simulink model "inverse_test"  (R2020b)
settings: Solver=VariableStepAuto  StartTime=0.0  StopTime=30  RelTol=1e-3
model workspace (MAT data in the model file):
  l1 = Simulink.Parameter
  l1.Value = 0.2
  l1.Description = '"Bicep length"'
  l1.DataType = 'auto'
  l1.Dimensions = [1 1]
  l2 = Simulink.Parameter
  l2.Value = 0.15
  l2.Description = '"Forearm length"'
  l2.DataType = 'auto'
  l2.Dimensions = [1 1]
libraries: pid_lib x2, simulink_extras x1
settings Model: PacingRate=0.500000  OrderedModelArguments=off  Creator=Luke Bidulka  LastModifiedBy=ndroz

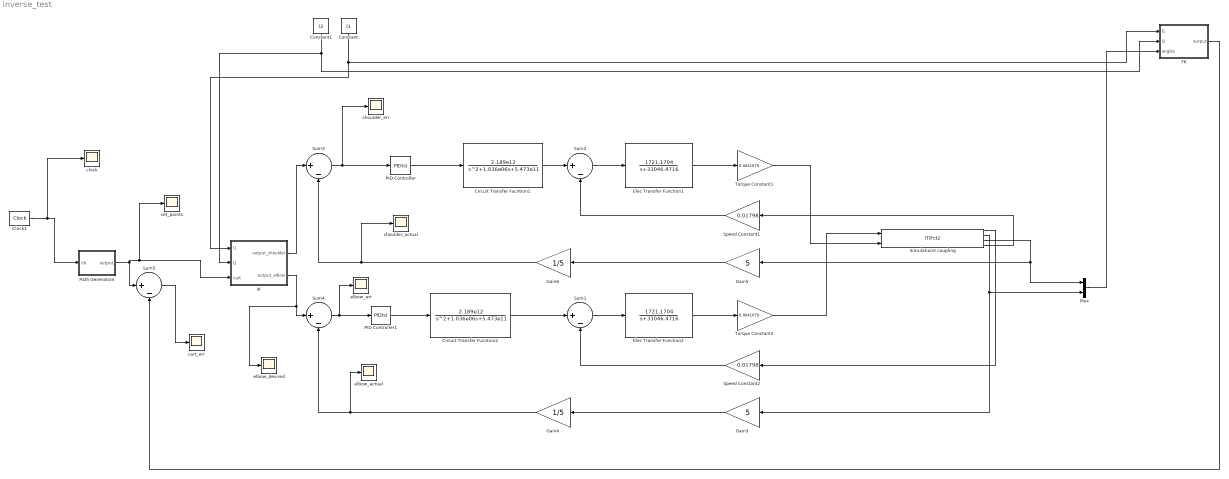
== system inverse_test ==
  Circuit Transfer Fucntion1 : TransferFcn  Numerator=[2.189e12]  Denominator=[1 1.036e06 5.473e11]
  Circuit Transfer Fucntion2 : TransferFcn  Numerator=[2.189e12]  Denominator=[1 1.036e06 5.473e11]
  Clock1 : simulink_extras/Flip Flops/Clock  period=0.01
  Constant : Constant  Value=l1
  Constant1 : Constant  Value=l2
  Elec Transfer Function1 : TransferFcn  Numerator=[1721.1704]  Denominator=[1 33046.4716]
  Elec Transfer Function2 : TransferFcn  Numerator=[1721.1704]  Denominator=[1 33046.4716]
  FK : MATLAB Function  TreatAsAtomicUnit=on
  Gain3 : Gain  Gain=5
  Gain4 : Gain  Gain=1/5
  Gain5 : Gain  Gain=5
  Gain6 : Gain  Gain=1/5
  IK : MATLAB Function  TreatAsAtomicUnit=on
  Mux : Mux  Inputs=2
  PID Controller : pid_lib/PID Controller  Controller=PID  Form=Parallel  TimeDomain=Continuous-time  UseExternalTs=off  SampleTime=-1  IntegratorMethod=Forward Euler  FilterMethod=Forward Euler  ControllerParametersSource=internal  P=0.1  I=0  D=150  UseFilter=on  N=280  TunerSelectOption=Transfer Function Based (PID Tuner App)  InitialConditionSource=internal  InitialConditionForIntegrator=0  InitialConditionForFilter=0  DifferentiatorICPrevScaledInput=0  ExternalReset=none  TrackingMode=off  Kt=1  LimitOutput=off  SatLimitsSource=internal  UpperSaturationLimit=inf  LowerSaturationLimit=-inf  LinearizeAsGain=on  AntiWindupMode=none  Kb=1  POutMin=[]  POutMax=[]  IOutMin=[]  IOutMax=[]  DOutMin=[]  DOutMax=[]  NOutMin=[]  NOutMax=[]  SumOutMin=[]  SumOutMax=[]  SaturationOutMin=[]  SaturationOutMax=[]  PParamMin=[]  PParamMax=[]  IParamMin=[]  IParamMax=[]  DParamMin=[]  DParamMax=[]  NParamMin=[]  NParamMax=[]  KbParamMin=[]  KbParamMax=[]  KtParamMin=[]  KtParamMax=[]  KbOutMin=[]  KbOutMax=[]  KtOutMin=[]  KtOutMax=[]  IntegratorOutMin=[]  IntegratorOutMax=[]  FilterOutMin=[]  FilterOutMax=[]  SumI1OutMin=[]  SumI1OutMax=[]  SumI2OutMin=[]  SumI2OutMax=[]  SumI3OutMin=[]  SumI3OutMax=[]  SumI4OutMin=[]  SumI4OutMax=[]  SumDOutMin=[]  SumDOutMax=[]  DifferentiatorOutMin=[]  DifferentiatorOutMax=[]  FilterDiffOutCoefMin=[]  FilterDiffOutCoefMax=[]  ReciprocalOutMin=[]  ReciprocalOutMax=[]  SumDenOutMin=[]  SumDenOutMax=[]  SumNumOutMin=[]  SumNumOutMax=[]  DivideOutMin=[]  DivideOutMax=[]  UdiffTsProdOutMin=[]  UdiffTsProdOutMax=[]  NTsProdOutMin=[]  NTsProdOutMax=[]  UintegralTsProdOutMin=[]  UintegralTsProdOutMax=[]  UngainTsProdOutMin=[]  UngainTsProdOutMax=[]  IntegratorContinuousStateAttributes=''  IntegratorStateMustResolveToSignalObject=off  IntegratorRTWStateStorageClass=Auto  FilterContinuousStateAttributes=''  FilterStateMustResolveToSignalObject=off  FilterRTWStateStorageClass=Auto  ParallelPVariant=InternalParameters  IdealPVariant=Disabled  IVariant=InternalParameters  DVariant=InternalParameters  IntegratorVariant=Continuous  SatVariant=Disabled  AWVariant=Passthrough  PCopyVariant=Disabled  TRVariant=Disabled  FdbkBlocksVariant=Forward  IdealPFdbkVariant=Disabled  SatFdbkVariant=Disabled  DerivativeFilterVariant=ContFilter  NVariant=InternalParameters  NCopyVariant=Disabled  FilterICVariant=InternalICsFilter  IntegratorICVariant=InternalICs  ExternalResetVariant=Disabled  TRSumVariant=Passthrough  SumFdbkVariant=Disabled  SumVariant=Sum_PID  TsampFilterVariant=InternalTs  TsampNgainVariant=Passthrough  TsampIntegralVariant=Passthrough  ExternalSaturationOutDataTypeStr=Inherit: Same as second input
  PID Controller1 : pid_lib/PID Controller  Controller=PID  Form=Parallel  TimeDomain=Continuous-time  UseExternalTs=off  SampleTime=-1  IntegratorMethod=Forward Euler  FilterMethod=Forward Euler  ControllerParametersSource=internal  P=100  I=50  D=300  UseFilter=on  N=280  TunerSelectOption=Transfer Function Based (PID Tuner App)  InitialConditionSource=internal  InitialConditionForIntegrator=0  InitialConditionForFilter=0  DifferentiatorICPrevScaledInput=0  ExternalReset=none  TrackingMode=off  Kt=1  LimitOutput=off  SatLimitsSource=internal  UpperSaturationLimit=inf  LowerSaturationLimit=-inf  LinearizeAsGain=on  AntiWindupMode=none  Kb=1  POutMin=[]  POutMax=[]  IOutMin=[]  IOutMax=[]  DOutMin=[]  DOutMax=[]  NOutMin=[]  NOutMax=[]  SumOutMin=[]  SumOutMax=[]  SaturationOutMin=[]  SaturationOutMax=[]  PParamMin=[]  PParamMax=[]  IParamMin=[]  IParamMax=[]  DParamMin=[]  DParamMax=[]  NParamMin=[]  NParamMax=[]  KbParamMin=[]  KbParamMax=[]  KtParamMin=[]  KtParamMax=[]  KbOutMin=[]  KbOutMax=[]  KtOutMin=[]  KtOutMax=[]  IntegratorOutMin=[]  IntegratorOutMax=[]  FilterOutMin=[]  FilterOutMax=[]  SumI1OutMin=[]  SumI1OutMax=[]  SumI2OutMin=[]  SumI2OutMax=[]  SumI3OutMin=[]  SumI3OutMax=[]  SumI4OutMin=[]  SumI4OutMax=[]  SumDOutMin=[]  SumDOutMax=[]  DifferentiatorOutMin=[]  DifferentiatorOutMax=[]  FilterDiffOutCoefMin=[]  FilterDiffOutCoefMax=[]  ReciprocalOutMin=[]  ReciprocalOutMax=[]  SumDenOutMin=[]  SumDenOutMax=[]  SumNumOutMin=[]  SumNumOutMax=[]  DivideOutMin=[]  DivideOutMax=[]  UdiffTsProdOutMin=[]  UdiffTsProdOutMax=[]  NTsProdOutMin=[]  NTsProdOutMax=[]  UintegralTsProdOutMin=[]  UintegralTsProdOutMax=[]  UngainTsProdOutMin=[]  UngainTsProdOutMax=[]  IntegratorContinuousStateAttributes=''  IntegratorStateMustResolveToSignalObject=off  IntegratorRTWStateStorageClass=Auto  FilterContinuousStateAttributes=''  FilterStateMustResolveToSignalObject=off  FilterRTWStateStorageClass=Auto  ParallelPVariant=InternalParameters  IdealPVariant=Disabled  IVariant=InternalParameters  DVariant=InternalParameters  IntegratorVariant=Continuous  SatVariant=Disabled  AWVariant=Passthrough  PCopyVariant=Disabled  TRVariant=Disabled  FdbkBlocksVariant=Forward  IdealPFdbkVariant=Disabled  SatFdbkVariant=Disabled  DerivativeFilterVariant=ContFilter  NVariant=InternalParameters  NCopyVariant=Disabled  FilterICVariant=InternalICsFilter  IntegratorICVariant=InternalICs  ExternalResetVariant=Disabled  TRSumVariant=Passthrough  SumFdbkVariant=Disabled  SumVariant=Sum_PID  TsampFilterVariant=InternalTs  TsampNgainVariant=Passthrough  TsampIntegralVariant=Passthrough  ExternalSaturationOutDataTypeStr=Inherit: Same as second input
  Path Generation : MATLAB Function  TreatAsAtomicUnit=on
  SimulationX coupling : S-Function  FunctionName=ITIFct2  Parameters=ip, port, ts, nIn, nOut  SFunctionDeploymentMode=off  EnableBusSupport=off  mask{ip='localhost', port=4098, ts=0.001, nIn=2, nOut=4}
      mask prompts: ip "Address: ip"; port "Port Number: port [-]"; ts "Communication Step Size: ts [s]"; nIn "Input Vector Dimension (to SimulationX): nIn [-]"; nOut "Output Vector Dimension (from SimulationX): nOut [-]"
      mask help: Coupling Element
  Speed Constant1 : Gain  Gain=0.01798
  Speed Constant2 : Gain  Gain=0.01798
  Sum{1..5} (5 alike) : Sum  Inputs=|+-
  Torque Constant1 : Gain  Gain=0.0041079
  Torque Constant2 : Gain  Gain=0.0041079
  cart_err : Scope
  clock : Scope
  elbow_actual : Scope
  elbow_desired : Scope
  elbow_err : Scope
  set_points : Scope
  shoulder_actual : Scope
  shoulder_err : Scope
  wires:
  Path Generation/1(output) -> set_points/1, IK/3(cart), Sum5/1
  Constant1/1 -> FK/2(l2), IK/2(l2)
  Constant/1 -> FK/1(l1), IK/1(l1)
  Gain5/1 -> Gain6/1
  Elec Transfer Function1/1 -> Torque Constant1/1
  Circuit Transfer Fucntion1/1 -> Sum2/1
  Speed Constant1/1 -> Sum2/2
  Sum2/1 -> Elec Transfer Function1/1
  Sum4/1 -> PID Controller1/1, elbow_err/1
  Elec Transfer Function2/1 -> Torque Constant2/1
  Speed Constant2/1 -> Sum1/2
  Gain3/1 -> Gain4/1
  Sum1/1 -> Elec Transfer Function2/1
  Circuit Transfer Fucntion2/1 -> Sum1/1
  Gain4/1 -> elbow_actual/1, Sum4/2
  IK/2(output_elbow) -> elbow_desired/1, Sum4/1
  Mux/1 -> FK/3(angles)
  Gain6/1 -> shoulder_actual/1, Sum3/2
  SimulationX coupling/1 -> Speed Constant2/1
  SimulationX coupling/2 -> Mux/2, Gain3/1
  SimulationX coupling/3 -> Mux/1, Gain5/1
  SimulationX coupling/4 -> Speed Constant1/1
  Torque Constant2/1 -> SimulationX coupling/1
  Torque Constant1/1 -> SimulationX coupling/2
  Sum3/1 -> PID Controller/1, shoulder_err/1
  PID Controller/1 -> Circuit Transfer Fucntion1/1
  PID Controller1/1 -> Circuit Transfer Fucntion2/1
  IK/1(output_shoulder) -> Sum3/1
  FK/1(output) -> Sum5/2
  Sum5/1 -> cart_err/1
  Clock1/1 -> clock/1, Path Generation/1(clk)

== matlab function inverse_test/FK ==
  data: l1 input; l2 input; angles input; output output
% Fwd Kinematics
function output = Fwd_Kin(l1, l2, angles)

    q0 = angles(1); % Configuration-space shoulder angle
    q1 = angles(2); % Configuration-space elbow angle

    % Get task-space coordinates
    x = l1*cos(q0) + l2*cos(q0+q1);
    y = l1*sin(q0) + l2*sin(q0+q1);

    % Output the task-space cartesian coordinats
    output = [x;y];

end

== matlab function inverse_test/IK ==
  data: l1 input; l2 input; cart input; output_shoulder output; output_elbow output
% Inv Kinematics
function [output_shoulder,output_elbow] = Inv_Kin(l1, l2, cart)
    x = cart(1); % Task-space x coord
    y = cart(2); % Task-space y coord
    
    % Get q1 first, need it to calculate q0. We will always
    % take the "right-handed" solution where q1 is (+). 
    q1 = abs(acos((x^2 + y^2 - l1^2 - l2^2)/(2*l1*l2)));

    % Get q0
    gamma = atan(y/x);
    beta = atan((l2*sin(q1))/(l1 + l2*cos(q1)));

    q0 = abs(gamma - beta);
    
    % Ouput our angle vector
    output_shoulder = q0;
    output_elbow = q1;
    
end

== matlab function inverse_test/Path Generation ==
  settings: sampleTime=0.2
  data: output output; clk input
function output = path_gen(clk)
    persistent count path_points path_size
    
    if isempty(count)
        count = 1;
        path_points = generate_path();
        path_size = length(path_points);
    end
    
    if clk == 1
        if count ~= path_size
            count = count + 1;
        end
    end
    
    output = path_points(count,:);
end

function output = generate_path()
    persistent count event event_count array_position x_value x_value_increment

    t = (0:0.1:10)'; % Time
    idle = 0;
    first_marsh = 1;
    first_marsh_idle = 2;
    second_marsh = 3;
    second_marsh_idle = 4;
    third_marsh = 5;
    third_marsh_idle = 6;
    garbage = 7;
    table_length = 0.3;
    table_angle = 50;
    table_origin = [0.13 0.25];
    
    current_point = [0 0]; %Initialize
    next_point = [0 0]; %Initialize
    starting_point = [0.2 0.15];
    first_marsh_point = [table_origin(1)-table_length/4*sind(table_angle) table_origin(2)+table_length/4*cosd(table_angle)];
    second_marsh_point = table_origin;
    third_marsh_point = [table_origin(1)+table_length/4*sind(table_angle) table_origin(2)-table_length/4*cosd(table_angle)];
    first_garbage_point = [first_marsh_point(1)-0.1*sind(90-table_angle) first_marsh_point(2)-0.1*cosd(90-table_angle)];
    second_garbage_point = [second_marsh_point(1)-0.1*sind(90-table_angle) second_marsh_point(2)-0.1*cosd(90-table_angle)];
    third_garbage_point = [third_marsh_point(1)-0.1*sind(90-table_angle) third_marsh_point(2)-0.1*cosd(90-table_angle)];

    path_vector = [garbage first_marsh_idle first_marsh garbage second_marsh_idle second_marsh garbage third_marsh_idle third_marsh garbage idle];
    path_points = zeros(100000,2);
    
    if isempty(count)
        event_count = 1;
        count = 1;
        array_position = 1;
        x_value_increment = 0.03;
    end
    
    while event_count <= length(path_vector)
        event = path_vector(event_count);
        x_value = 4.6;

        switch event
            case garbage 
                if event_count == 1
                    current_point = starting_point;
                    next_point = second_garbage_point;
                elseif path_vector(event_count - 1) == first_marsh
                    current_point = first_marsh_point;
                    next_point = first_garbage_point;
                elseif path_vector(event_count - 1) == second_marsh
                    current_point = second_marsh_point;
                    next_point = second_garbage_point;
                else 
                    current_point = third_marsh_point;
                    next_point = third_garbage_point;
                end
            case first_marsh_idle
                current_point = second_garbage_point;
                next_point = first_garbage_point;
            case first_marsh
                current_point = first_garbage_point;
                next_point = first_marsh_point;
            case second_marsh_idle
                current_point = first_garbage_point;
                next_point = second_garbage_point;    
            case second_marsh 
                current_point = second_garbage_point;
                next_point = second_marsh_point;
            case third_marsh_idle
                current_point = second_garbage_point;
                next_point = third_garbage_point; 
            case third_marsh
                current_point = third_garbage_point;
                next_point = third_marsh_point;
            case idle
                current_point = third_garbage_point;
                next_point = second_garbage_point;
        end

        x_point = current_point(1);
        y_point = current_point(2);
        

        while ((abs(x_point - current_point(1)) <= abs(next_point(1) - current_point(1))) && (abs(y_point - current_point(2)) <= abs(next_point(2) - current_point(2))))
            if (event == first_marsh || event == second_marsh || event == third_marsh)
                increment_x = (next_point(1) - current_point(1)) / (1*(x_value^3));
                increment_y = (next_point(2) - current_point(2)) / (1*(x_value^3));
                if (1*(x_value^3) < 500)
                    x_value = x_value + x_value_increment;
                end
            else
                increment_x = (next_point(1) - current_point(1)) / length(t);
                increment_y = (next_point(2) - current_point(2)) / length(t);
            end
            x_point = x_point + increment_x;
            y_point = y_point + increment_y;
            path_points(array_position,:) = [x_point y_point];
            array_position = array_position + 1;
        end   

        for i = 1:75
            path_points(array_position,:) = [x_point y_point];
            array_position = array_position + 1;
        end

        event_count = event_count +1;
    end
    
    path_points(array_position:end, :) = [];
    output = path_points;
end
